simulink model "LQG_2by2_2workspace"  (Simulink 10.2)
settings: Solver=FixedStepDiscrete  StartTime=0.0  StopTime=300  FixedStep=h  RelTol=1e-3  EnableMultiTasking=on
values from neighbouring files (symbols this model uses):
  Ad = sysd.a    [LQG_2by2_sim.m]
  Bd = sysd.b    [LQG_2by2_sim.m]
  C = sysd.c    [LQG_2by2_sim.m]
  h = 0.01    [LQG_2by2_sim.m]
  K = (4-3*rho+q)./(8+10*rho+2*q)    [kalman_example.m]
  K_FF = inv(C*inv(eye(2)-Ad+Bd*L)*Bd)    [LQG_2by2_sim.m]
  R1 = diag([0.1 0.05])    [LQG_2by2_sim.m]    (also in kalman_example.m = 0.05)
  R2 = 0.1*eye(2)    [LQG_2by2_sim.m]
undefined symbols (not defined in the file or in its folder): L
settings Model: Creator=tw  LastModifiedBy=tw
settings DataIOCC: LimitDataPoints=on  MaxDataPoints=1000000
settings OptimizationCC: ExpressionDepthLimit=2147483647  InitFltsAndDblsToZero=on
settings DebuggingCC: SaveWithParameterizedLinksMsg=none  SolverPrmCheckMsg=warning  StateNameClashWarn=warning
settings GRTTargetCC: TargetFcnLib=ansi_tfl_tmw.mat

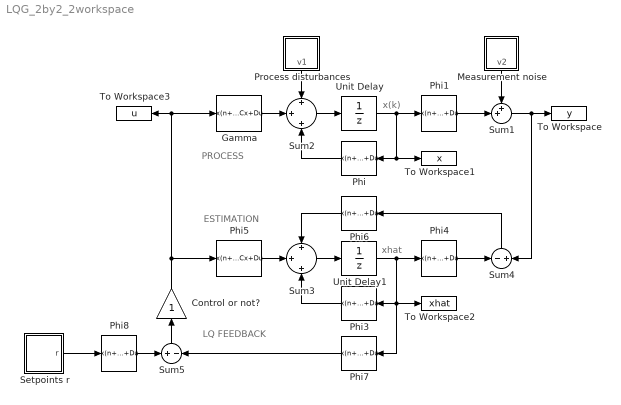
== system LQG_2by2_2workspace ==
  note: x(k)
  note: xhat
  note: PROCESS
  note: LQ FEEDBACK
  note: ESTIMATION
  Control or not? : Gain
  Gamma : DiscreteStateSpace  A=[]  B=[]  C=[]  D=Bd  SampleTime=-1  mask(Vector gain){}
      mask Display: disp('Bd')
  Measurement noise : Subsystem
  Phi : DiscreteStateSpace  A=[]  B=[]  C=[]  D=Ad  SampleTime=-1  mask(Vector gain){}
      mask Display: disp('Ad')
  Phi1 : DiscreteStateSpace  A=[]  B=[]  C=[]  D=C  SampleTime=-1  mask(Vector gain){}
      mask Display: disp('C')
  Phi3 : DiscreteStateSpace  A=[]  B=[]  C=[]  D=Ad  SampleTime=-1  mask(Vector gain){}
      mask Display: disp('Ad')
  Phi4 : DiscreteStateSpace  A=[]  B=[]  C=[]  D=C  SampleTime=-1  mask(Vector gain){}
      mask Display: disp('C')
  Phi5 : DiscreteStateSpace  A=[]  B=[]  C=[]  D=Bd  SampleTime=-1  mask(Vector gain){}
      mask Display: disp('Bd')
  Phi6 : DiscreteStateSpace  A=[]  B=[]  C=[]  D=K  SampleTime=-1  mask(Vector gain){}
      mask Display: disp('K')
  Phi7 : DiscreteStateSpace  A=[]  B=[]  C=[]  D=L  SampleTime=-1  mask(Vector gain){}
      mask Display: disp('L')
  Phi8 : DiscreteStateSpace  A=[]  B=[]  C=[]  D=K_FF  SampleTime=-1  mask(Vector gain){}
      mask Display: disp('K_FF')
  Process disturbances : Subsystem
  Setpoints r : Subsystem
  Sum1 : Sum  Inputs=++|
  Sum2 : Sum  Inputs=+|+|+
  Sum3 : Sum  Inputs=+|+|+
  Sum4 : Sum  Inputs=-|+
  Sum5 : Sum  Inputs=+|-
  To Workspace : ToWorkspace  VariableName=y  SampleTime=-1
  To Workspace1 : ToWorkspace  VariableName=x  SampleTime=-1
  To Workspace2 : ToWorkspace  VariableName=xhat  SampleTime=-1
  To Workspace3 : ToWorkspace  VariableName=u  SampleTime=-1
  Unit Delay : UnitDelay  SampleTime=-1  HasFrameUpgradeWarning=on
  Unit Delay1 : UnitDelay  SampleTime=-1  HasFrameUpgradeWarning=on
  wires:
  Sum2/1 -> Unit Delay/1
  Unit Delay/1 -> Phi1/1, Phi/1, To Workspace1/1
  Phi1/1 -> Sum1/2
  Sum1/1 -> Sum4/2, To Workspace/1
  Measurement noise/1(v2) -> Sum1/1
  Process disturbances/1(v1) -> Sum2/1
  Gamma/1 -> Sum2/2
  Phi/1 -> Sum2/3
  Sum3/1 -> Unit Delay1/1
  Unit Delay1/1 -> Phi4/1, Phi3/1, To Workspace2/1, Phi7/1
  Phi5/1 -> Sum3/2
  Phi3/1 -> Sum3/3
  Phi4/1 -> Sum4/1
  Sum4/1 -> Phi6/1
  Phi6/1 -> Sum3/1
  Phi7/1 -> Sum5/2
  Sum5/1 -> Control or not?/1
  Phi8/1 -> Sum5/1
  Control or not?/1 -> Phi5/1, Gamma/1, To Workspace3/1
  Setpoints r/1(r) -> Phi8/1

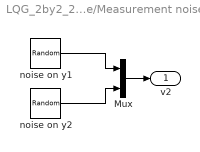
== system LQG_2by2_2workspace/Measurement noise ==
  Mux : Mux  Inputs=2
  noise on y1 : RandomNumber  Variance=R2(1,1)  Seed=5  SampleTime=h
  noise on y2 : RandomNumber  Variance=R2(2,2)  Seed=4  SampleTime=h
  v2 : Outport
  wires:
  noise on y1/1 -> Mux/1
  noise on y2/1 -> Mux/2
  Mux/1 -> v2/1

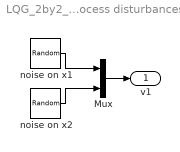
== system LQG_2by2_2workspace/Process disturbances ==
  Mux : Mux  Inputs=2
  noise on x1 : RandomNumber  Variance=R1(1,1)  Seed=3  SampleTime=h
  noise on x2 : RandomNumber  Variance=R1(2,2)  Seed=2  SampleTime=h
  v1 : Outport
  wires:
  noise on x1/1 -> Mux/1
  noise on x2/1 -> Mux/2
  Mux/1 -> v1/1

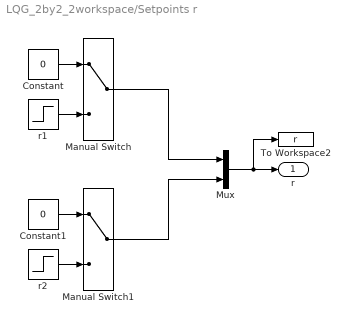
== system LQG_2by2_2workspace/Setpoints r ==
  Constant : Constant  Value=0
  Constant1 : Constant  Value=0
  Manual Switch : ManualSwitch
  Manual Switch1 : ManualSwitch
  Mux : Mux  Inputs=2
  To Workspace2 : ToWorkspace  VariableName=r  SampleTime=-1
  r1 : Step  After=4  SampleTime=h
  r2 : Step  Time=5  After=4  SampleTime=h
  r : Outport
  wires:
  Mux/1 -> r/1, To Workspace2/1
  r1/1 -> Manual Switch/2
  Manual Switch/1 -> Mux/1
  Constant/1 -> Manual Switch/1
  Constant1/1 -> Manual Switch1/1
  r2/1 -> Manual Switch1/2
  Manual Switch1/1 -> Mux/2
